simulink model "Total_B2B"  (R2018a)
settings: Solver=ode8  StartTime=0.0  StopTime=10  FixedStep=20e-6  RelTol=1e-3
values from neighbouring files (symbols this model uses):
  A = R^2*pi    (= 24996.5217713)    [Total_init.m]    (also in Total_init_trafo.m)
  C1 = 0.0117    [Total_init.m]    (also in Total_init_trafo.m)
  C2 = 5500    [Total_init.m]    (also in Total_init_trafo.m)
  C3 = 10    [Total_init.m]    (also in Total_init_trafo.m)
  C4 = 0    [Total_init.m]    (also in Total_init_trafo.m)
  C5 = 160    [Total_init.m]    (also in Total_init_trafo.m)
  C6 = 23.38    [Total_init.m]    (also in Total_init_trafo.m)
  C_dc = 1e-2    (= 0.01)    [Total_init.m]    (also in Total_init_trafo.m)
  Cx = 0    [Total_init.m]    (also in Total_init_trafo.m)
  Ir = 2*Pr/(3*Er*cosphi)    (= 2057.61316872)    [Total_init.m]    (also in Total_init_trafo.m)
  J = 12.8e6    (= 12800000)    [Total_init.m]    (also in Total_init_trafo.m)
  Jr = 3*m*r^2    (= 105248711.1)    [Total_init.m]    (also in Total_init_trafo.m)
  KI_d = KP_d*Rs/Ld    (= 1454)    [Total_init.m]    (also in Total_init_trafo.m)
  KP_d = 50    [Total_init.m]    (also in Total_init_trafo.m)
  KP_g = 5    [Total_init.m]    (also in Total_init_trafo.m)
  KP_gv = 5    [Total_init.m]    (also in Total_init_trafo.m)
  lambda_m = Er/(om_r*p)    (= 21.4859173174)    [Total_init.m]    (also in Total_init_trafo.m)
  lambda_opt = 9.35    [Total_init.m]    (also in Total_init_trafo.m)
  Ld = 0.005    [Total_init.m]    (also in Total_init_trafo.m)
  Lg = 1e-3    (= 0.001)    [Total_init.m]    (also in Total_init_trafo.m)
  Linvmat = Lmat^(-1)    [Total_init.m]    (also in Total_init_trafo.m)
  Lq = 0.005    [Total_init.m]    (also in Total_init_trafo.m)
  om0 = om_r    (= 1.0471975512)    [Total_init.m]    (also in Total_init_trafo.m)
  om_g = 100*pi    (= 314.159265359)    [Total_init.m]    (also in Total_init_trafo.m)
  om_r = 10/60*2*pi    (= 1.0471975512)    [Total_init.m]    (also in Total_init_trafo.m)
  p = 160    [Total_init.m]    (also in Total_init_trafo.m)
  Pr = 10e6    (= 10000000)    [Total_init.m]    (also in Total_init_trafo.m)
  psi0 = Lmat*I0'+psif    [Total_init.m]    (also in Total_init_trafo.m)
  psif = [lambda_m; 0]    [Total_init.m]    (also in Total_init_trafo.m)
  R = 89.2    [Total_init.m]    (also in Total_init_trafo.m)
  R_cs = 1e9    (= 1000000000)    [Total_init.m]    (also in Total_init_trafo.m)
  R_dc = 1e-3    (= 0.001)    [Total_init.m]    (also in Total_init_trafo.m)
  Rg = 1e-6    (= 1e-06)    [Total_init.m]    (also in Total_init_trafo.m)
  rho = 1.225    [Total_init.m]    (also in Total_init_trafo.m)
  Rmat = [Rs 0;         0 Rs]    [Total_init.m]    (also in Total_init_trafo.m)
  Rs = 0.1454    [Total_init.m]    (also in Total_init_trafo.m)
  ts = 0.0001    [Total_init.m]    (also in Total_init_trafo.m)
  Vac = 4000    [Total_init.m]    (also in Total_init_trafo.m)
  Vdc = Vac*sqrt(3)    [Total_init.m]    (also in Total_init_trafo.m)
  Vgsc = Vac    (= 4000)    [Total_init.m]    (also in Total_init_trafo.m)
libraries: powerlib x17, simulink x9
(part 1 of 2)
settings Model: Creator=chiel  LastModifiedBy=chiel
settings CodeAppCC: StateflowObjectComments=on

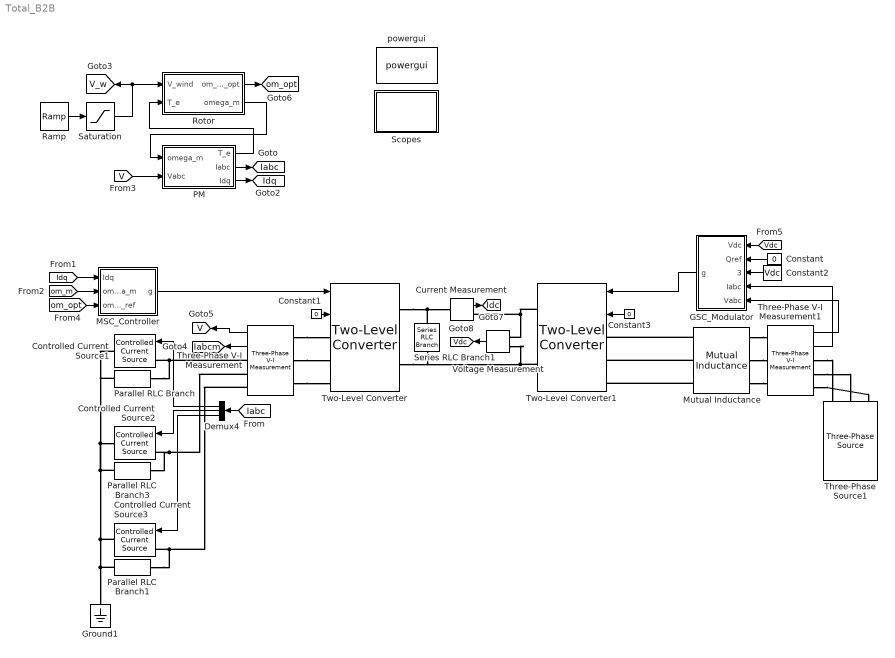
== system Total_B2B ==
  Constant : Constant  Value=0
  Constant1 : Constant  Value=0
  Constant2 : Constant  Value=Vdc
  Constant3 : Constant  Value=0
  Controlled Current Source1 : powerlib/Electrical Sources/Controlled Current Source  Initialize=on  Source_Type=AC  Amplitude=0  Phase=0  Frequency=0  Measurements=None
  Controlled Current Source2 : powerlib/Electrical Sources/Controlled Current Source  Initialize=on  Source_Type=AC  Amplitude=0  Phase=0  Frequency=0  Measurements=None
  Controlled Current Source3 : powerlib/Electrical Sources/Controlled Current Source  Initialize=on  Source_Type=AC  Amplitude=0  Phase=0  Frequency=0  Measurements=None
  Current Measurement : powerlib/Measurements/Current Measurement  PhasorSimulation=off  OutputType=Complex  PSBequivalent=0
  Demux4 : Demux  Outputs=3
  GSC_Modulator : Subsystem
  Ground1 : powerlib/Elements/Ground  LConnTagsString=a
  MSC_Controller : Subsystem
  Mutual Inductance : powerlib/Elements/Mutual Inductance  LConnTagsString=a|b|c  RConnTagsString=A|B|C  TypeOfMutual=Two or three windings with equal mutual terms  NumberOfWindings=3  SelfImpedance1=[Rg Lg]  SelfImpedance2=[Rg Lg]  ThreeWindings=on  SelfImpedance3=[Rg Lg]  MutualImpedance=[0 0]  InductanceMatrix="[1.0 0.9  0.9 ;  0.9 1.0  0.9;  0.9 0.9 1.0 ] * 1e-3"  ResistanceMatrix="[1.0 0.9  0.9 ;  0.9 1.0  0.9;  0.9 0.9 1.0 ]"  Measurements=None
      settings: AttributesFormatString=\n  SourceProductName=Simscape Power Systems  SourceProductBaseCode=PS
  PM : Subsystem
  Parallel RLC Branch : powerlib/Elements/Parallel RLC Branch  LConnTagsString=a  RConnTagsString=__new0  BranchType=R  Resistance=R_cs  Inductance=Lg  SetiL0=off  InitialCurrent=0  Capacitance=1e-6  Setx0=off  InitialVoltage=0  Measurements=None
  Parallel RLC Branch1 : powerlib/Elements/Parallel RLC Branch  LConnTagsString=a  RConnTagsString=__new0  BranchType=R  Resistance=R_cs  Inductance=Lg  SetiL0=off  InitialCurrent=0  Capacitance=1e-6  Setx0=off  InitialVoltage=0  Measurements=None
  Parallel RLC Branch3 : powerlib/Elements/Parallel RLC Branch  LConnTagsString=a  RConnTagsString=__new0  BranchType=R  Resistance=R_cs  Inductance=Lg  SetiL0=off  InitialCurrent=0  Capacitance=1e-6  Setx0=off  InitialVoltage=0  Measurements=None
  Ramp : simulink/Sources/Ramp  slope=0.5  start=0  InitialOutput=15
  Rotor : Subsystem
  Saturation : Saturate  UpperLimit=15
  Scopes : Subsystem
  Series RLC Branch1 : powerlib/Elements/Series RLC Branch  LConnTagsString=__new0  RConnTagsString=__new0  BranchType=RC  Resistance=R_dc  Inductance=1e-3  SetiL0=off  InitialCurrent=0  Capacitance=C_dc  Setx0=on  InitialVoltage=Vdc  Measurements=None
  Three-Phase V-I Measurement : powerlib/Measurements/Three-Phase V-I Measurement  VoltageMeasurement=phase-to-ground  SetLabelV=off  LabelV=Vabc  Vpu=off  VpuLL=off  CurrentMeasurement=yes  SetLabelI=off  LabelI=Iabc  Ipu=off  Pbase=100e6  Vbase=500e3  OutputType=Complex  PhasorSimulation=off  PSBequivalent=0
  Three-Phase V-I Measurement1 : powerlib/Measurements/Three-Phase V-I Measurement  VoltageMeasurement=phase-to-ground  SetLabelV=off  LabelV=Vabc  Vpu=off  VpuLL=off  CurrentMeasurement=yes  SetLabelI=off  LabelI=Iabc  Ipu=off  Pbase=100e6  Vbase=500e3  OutputType=Complex  PhasorSimulation=off  PSBequivalent=0
  Three-Phase Source1 : powerlib/Electrical Sources/Three-Phase Source  InternalConnection=Yg  VoltagePhases=off  Voltage=Vgsc/sqrt(2)*sqrt(3)  PhaseAngle=90  Voltage_phases=[25e3 25e3 25e3]/sqrt(3)  PhaseAngles_phases=[0 -120 +120]  Frequency=50  NonIdealSource=on  SpecifyImpedance=off  Resistance=1e-9  Inductance=1e-12  ShortCircuitLevel=100e6  BaseVoltage=Vgsc/sqrt(2)*sqrt(3)  XRratio=7  BusType=swing  Pref=10e3  Qref=0  Prefabc=[10e3, 10e3, 10e3]  Qrefabc=[0, 0, 0]  Qmin=-inf  Qmax=inf
  Two-Level Converter : powerlib/Power Electronics/Two-Level Converter  ModelType=Switching devices  Ron=1e-3  Rs=1e6  Cs=inf  Vforward=[0,0]  Ron_Diode=1e-3  Rs_Diode=1e6  Cs_Diode=inf  Vf_Diode=1e-3  Rs_CurrentSource=inf
      settings: SourceProductName=Simscape Power Systems  SourceProductBaseCode=PS
  Two-Level Converter1 : powerlib/Power Electronics/Two-Level Converter  ModelType=Switching function  Ron=1e-3  Rs=1e6  Cs=inf  Vforward=[0,0]  Ron_Diode=1e-3  Rs_Diode=1e6  Cs_Diode=inf  Vf_Diode=1e-3  Rs_CurrentSource=inf
      settings: SourceProductName=Simscape Power Systems  SourceProductBaseCode=PS
  Voltage Measurement : powerlib/Measurements/Voltage Measurement  PhasorSimulation=off  OutputType=Complex  PSBequivalent=0
  powergui : powerlib/powergui  Priority=1  SimulationMode=Discrete  SampleTime=20e-6  frequency=60  Iterations=50  frequencyindice=0  Pbase=100e6  ErrMax=1e-4  UnitsV=kV  UnitsW=MW  buscounter=0  FunctionMessages=off  echomessages=off  EnableUseOfTLC=off  CurrentSourceSwitches=off  DisableSnubberDevices=off  DisableRonSwitches=off  DisableVfSwitches=off  DisplayEquations=off  SolverType=Tustin/Backward Euler (TBE)  Interpol=off  ExternalGateDelay=off  methode=off  Ts=100  x0status=blocks  SPID=off  SwTol=0  HookPort=off  RestoreLinks=warning  ResistiveCurrentMeasurement=off  Frange=[0:2:500]  Ylog=off  Xlog=on  ShowGrid=off  save=off  variable=ZData  structure=0  ZoomFFT=off  StartTime=0.0  cycles=1  DisplayStyle=1  fundamental=60  FreqAxis=off  MaxFrequency=1000  frequencyindicesteady=1  RmsSteady=1  display=off
  tag scope: Iabc=global, Iabcm=global, Idc=global, Idq=global, V=global, V_w=global, Vdc=global, om_opt=global
  wires:
  [om_m] -> MSC_Controller/2(omega_m)
  [V] -> PM/2(Vabc)
  PM/2(Iabc) -> [Iabc]
  [Idq] -> MSC_Controller/1(Idq)
  PM/3(Idq) -> [Idq]
  Rotor/1(om_m_opt) -> [om_opt]
  [om_opt] -> MSC_Controller/3(omega_ref)
  Ramp/1 -> Saturation/1
  Saturation/1 -> Rotor/1(V_wind), [V_w]
  Three-Phase V-I Measurement/1 -> [V]
  Demux4/3 -> Controlled Current Source3/1
  Current Measurement/1 -> [Idc]
  Three-Phase V-I Measurement/2 -> [Iabcm]
  Constant1/1 -> Two-Level Converter/2
  Demux4/1 -> Controlled Current Source1/1
  Demux4/2 -> Controlled Current Source2/1
  [Iabc] -> Demux4/1
  Voltage Measurement/1 -> [Vdc]
  MSC_Controller/1(g) -> Two-Level Converter/1
  GSC_Modulator/1(g) -> Two-Level Converter1/1
  Constant3/1 -> Two-Level Converter1/2
  Constant/1 -> GSC_Modulator/2(Qref)
  [Vdc] -> GSC_Modulator/1(Vdc)
  Constant2/1 -> GSC_Modulator/3(Vdc_ref)
  Three-Phase V-I Measurement1/1 -> GSC_Modulator/5(Vabc)
  Three-Phase V-I Measurement1/2 -> GSC_Modulator/4(Iabc)
  Rotor/2(omega_m) -> PM/1(omega_m)
  PM/1(T_e) -> Rotor/2(T_e)
  connections:
  Controlled Current Source1/RConn1 -- Parallel RLC Branch/LConn1 -- Controlled Current Source2/RConn1 -- Parallel RLC Branch3/LConn1 -- Controlled Current Source3/RConn1 -- Ground1/LConn1 -- Parallel RLC Branch1/LConn1
  Series RLC Branch1/LConn1 -- Two-Level Converter/RConn1 -- Current Measurement/LConn1
  Voltage Measurement/LConn2 -- Two-Level Converter/RConn2 -- Series RLC Branch1/RConn1 -- Two-Level Converter1/RConn2
  Two-Level Converter1/RConn1 -- Current Measurement/RConn1 -- Voltage Measurement/LConn1
  Three-Phase V-I Measurement/LConn2 -- Two-Level Converter/LConn2
  Three-Phase V-I Measurement/RConn1 -- Parallel RLC Branch/RConn1 -- Controlled Current Source1/LConn1
  Three-Phase V-I Measurement/RConn2 -- Parallel RLC Branch3/RConn1 -- Controlled Current Source2/LConn1
  Three-Phase V-I Measurement/LConn3 -- Two-Level Converter/LConn3
  Three-Phase V-I Measurement/LConn1 -- Two-Level Converter/LConn1
  Three-Phase V-I Measurement/RConn3 -- Parallel RLC Branch1/RConn1 -- Controlled Current Source3/LConn1
  Three-Phase V-I Measurement1/RConn2 -- Three-Phase Source1/RConn2
  Three-Phase V-I Measurement1/RConn3 -- Three-Phase Source1/RConn3
  Three-Phase V-I Measurement1/RConn1 -- Three-Phase Source1/RConn1
  Mutual Inductance/LConn1 -- Two-Level Converter1/LConn1
  Mutual Inductance/LConn2 -- Two-Level Converter1/LConn2
  Mutual Inductance/LConn3 -- Two-Level Converter1/LConn3
  Mutual Inductance/RConn1 -- Three-Phase V-I Measurement1/LConn1
  Mutual Inductance/RConn2 -- Three-Phase V-I Measurement1/LConn2
  Mutual Inductance/RConn3 -- Three-Phase V-I Measurement1/LConn3

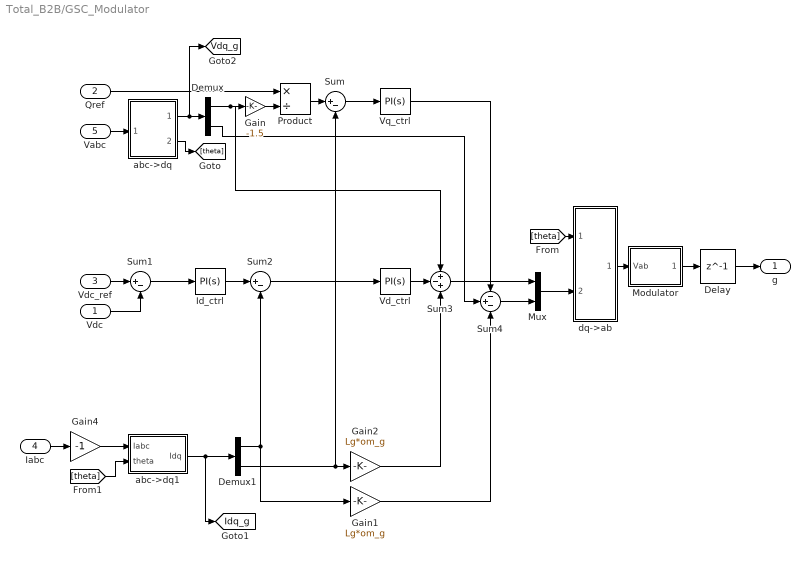
== system Total_B2B/GSC_Modulator ==
  Vdc : Inport
  Qref : Inport  Port=2
  Vdc_ref : Inport  Port=3
  Iabc : Inport  Port=4
  Vabc : Inport  Port=5
  Delay : Delay  DelayLength=1
  Demux : Demux  Outputs=2
  Demux1 : Demux  Outputs=2
  Gain : Gain  Gain=-1.5
  Gain1 : Gain  Gain=Lg*om_g
  Gain2 : Gain  Gain=Lg*om_g
  Gain4 : Gain  Gain=-1
  Id_ctrl : simulink/Continuous/PID Controller  Controller=PI  TimeDomain=Continuous-time  SampleTime=-1  IntegratorMethod=Forward Euler  FilterMethod=Forward Euler  Form=Parallel  UseFilter=on  ControllerParametersSource=internal  P=KP_gv  I=0  D=0  N=100  InitialConditionSource=internal  InitialConditionForIntegrator=0  InitialConditionForFilter=0  ExternalReset=none  LimitOutput=on  UpperSaturationLimit=Ir  LowerSaturationLimit=-Ir  LinearizeAsGain=on  AntiWindupMode=clamping  Kb=1  TrackingMode=off  Kt=1  PParamMin=[]  PParamMax=[]  IParamMin=[]  IParamMax=[]  DParamMin=[]  DParamMax=[]  NParamMin=[]  NParamMax=[]  KbParamMin=[]  KbParamMax=[]  KtParamMin=[]  KtParamMax=[]  POutMin=[]  POutMax=[]  IOutMin=[]  IOutMax=[]  DOutMin=[]  DOutMax=[]  NOutMin=[]  NOutMax=[]  KbOutMin=[]  KbOutMax=[]  KtOutMin=[]  KtOutMax=[]  IntegratorOutMin=[]  IntegratorOutMax=[]  FilterOutMin=[]  FilterOutMax=[]  SumOutMin=[]  SumOutMax=[]  SumI1OutMin=[]  SumI1OutMax=[]  SumI2OutMin=[]  SumI2OutMax=[]  SumI3OutMin=[]  SumI3OutMax=[]  SumDOutMin=[]  SumDOutMax=[]  SaturationOutMin=[]  SaturationOutMax=[]  IntegratorContinuousStateAttributes=''  IntegratorStateMustResolveToSignalObject=off  IntegratorRTWStateStorageClass=Auto  FilterContinuousStateAttributes=''  FilterStateMustResolveToSignalObject=off  FilterRTWStateStorageClass=Auto  DifferentiatorICPrevScaledInput=0  DifferentiatorOutMin=[]  DifferentiatorOutMax=[]  FilterDiffOutCoefMin=[]  FilterDiffOutCoefMax=[]  SumDenOutMin=[]  SumDenOutMax=[]  SumNumOutMin=[]  SumNumOutMax=[]  ReciprocalOutMin=[]  ReciprocalOutMax=[]  DivideOutMin=[]  DivideOutMax=[]  TunerSelectOption=Transfer Function Based (PID Tuner App)
  Modulator : Subsystem  mask{Fs=1/ts}
      mask prompts: Fs "Switching Frequency"
      mask DialogControl DescGroupVar Prompt: Swiching Parameters
  Mux : Mux  Inputs=2
  Product : Product  Inputs=*/
  Sum : Sum  Inputs=|+-
  Sum1 : Sum  Inputs=|+-
  Sum2 : Sum  Inputs=|+-
  Sum3 : Sum  Inputs=+-+
  Sum4 : Sum  Inputs=-+-
  Vd_ctrl : simulink/Continuous/PID Controller  Controller=PI  TimeDomain=Continuous-time  SampleTime=-1  IntegratorMethod=Forward Euler  FilterMethod=Forward Euler  Form=Parallel  UseFilter=on  ControllerParametersSource=internal  P=KP_g  I=0  D=0  N=100  InitialConditionSource=internal  InitialConditionForIntegrator=0  InitialConditionForFilter=0  ExternalReset=none  LimitOutput=on  UpperSaturationLimit=Vgsc  LowerSaturationLimit=-Vgsc  LinearizeAsGain=on  AntiWindupMode=clamping  Kb=1  TrackingMode=off  Kt=1  PParamMin=[]  PParamMax=[]  IParamMin=[]  IParamMax=[]  DParamMin=[]  DParamMax=[]  NParamMin=[]  NParamMax=[]  KbParamMin=[]  KbParamMax=[]  KtParamMin=[]  KtParamMax=[]  POutMin=[]  POutMax=[]  IOutMin=[]  IOutMax=[]  DOutMin=[]  DOutMax=[]  NOutMin=[]  NOutMax=[]  KbOutMin=[]  KbOutMax=[]  KtOutMin=[]  KtOutMax=[]  IntegratorOutMin=[]  IntegratorOutMax=[]  FilterOutMin=[]  FilterOutMax=[]  SumOutMin=[]  SumOutMax=[]  SumI1OutMin=[]  SumI1OutMax=[]  SumI2OutMin=[]  SumI2OutMax=[]  SumI3OutMin=[]  SumI3OutMax=[]  SumDOutMin=[]  SumDOutMax=[]  SaturationOutMin=[]  SaturationOutMax=[]  IntegratorContinuousStateAttributes=''  IntegratorStateMustResolveToSignalObject=off  IntegratorRTWStateStorageClass=Auto  FilterContinuousStateAttributes=''  FilterStateMustResolveToSignalObject=off  FilterRTWStateStorageClass=Auto  DifferentiatorICPrevScaledInput=0  DifferentiatorOutMin=[]  DifferentiatorOutMax=[]  FilterDiffOutCoefMin=[]  FilterDiffOutCoefMax=[]  SumDenOutMin=[]  SumDenOutMax=[]  SumNumOutMin=[]  SumNumOutMax=[]  ReciprocalOutMin=[]  ReciprocalOutMax=[]  DivideOutMin=[]  DivideOutMax=[]  TunerSelectOption=Transfer Function Based (PID Tuner App)
  Vq_ctrl : simulink/Continuous/PID Controller  Controller=PI  TimeDomain=Continuous-time  SampleTime=-1  IntegratorMethod=Forward Euler  FilterMethod=Forward Euler  Form=Parallel  UseFilter=on  ControllerParametersSource=internal  P=KP_g  I=0  D=0  N=100  InitialConditionSource=internal  InitialConditionForIntegrator=0  InitialConditionForFilter=0  ExternalReset=none  LimitOutput=on  UpperSaturationLimit=Vgsc  LowerSaturationLimit=-Vgsc  LinearizeAsGain=on  AntiWindupMode=none  Kb=1  TrackingMode=off  Kt=1  PParamMin=[]  PParamMax=[]  IParamMin=[]  IParamMax=[]  DParamMin=[]  DParamMax=[]  NParamMin=[]  NParamMax=[]  KbParamMin=[]  KbParamMax=[]  KtParamMin=[]  KtParamMax=[]  POutMin=[]  POutMax=[]  IOutMin=[]  IOutMax=[]  DOutMin=[]  DOutMax=[]  NOutMin=[]  NOutMax=[]  KbOutMin=[]  KbOutMax=[]  KtOutMin=[]  KtOutMax=[]  IntegratorOutMin=[]  IntegratorOutMax=[]  FilterOutMin=[]  FilterOutMax=[]  SumOutMin=[]  SumOutMax=[]  SumI1OutMin=[]  SumI1OutMax=[]  SumI2OutMin=[]  SumI2OutMax=[]  SumI3OutMin=[]  SumI3OutMax=[]  SumDOutMin=[]  SumDOutMax=[]  SaturationOutMin=[]  SaturationOutMax=[]  IntegratorContinuousStateAttributes=''  IntegratorStateMustResolveToSignalObject=off  IntegratorRTWStateStorageClass=Auto  FilterContinuousStateAttributes=''  FilterStateMustResolveToSignalObject=off  FilterRTWStateStorageClass=Auto  DifferentiatorICPrevScaledInput=0  DifferentiatorOutMin=[]  DifferentiatorOutMax=[]  FilterDiffOutCoefMin=[]  FilterDiffOutCoefMax=[]  SumDenOutMin=[]  SumDenOutMax=[]  SumNumOutMin=[]  SumNumOutMax=[]  ReciprocalOutMin=[]  ReciprocalOutMax=[]  DivideOutMin=[]  DivideOutMax=[]  TunerSelectOption=Transfer Function Based (PID Tuner App)
  abc->dq : Subsystem
  abc->dq1 : Subsystem
  dq->ab : Subsystem
  g : Outport
  tag scope: Idq_g=global, Vdq_g=global
  wires:
  Vabc/1 -> abc->dq/1(Vabc)
  Iabc/1 -> Gain4/1
  abc->dq/1(Vdq) -> [Vdq_g], Demux/1
  abc->dq1/1(Idq) -> [Idq_g], Demux1/1
  Gain/1 -> Product/2
  Qref/1 -> Product/1
  Demux1/2 -> Gain2/1, Sum/2
  Vdc/1 -> Sum1/2
  Sum1/1 -> Id_ctrl/1
  Demux1/1 -> Sum2/2, Gain1/1
  Vd_ctrl/1 -> Sum3/2
  Vq_ctrl/1 -> Sum4/1
  Mux/1 -> dq->ab/2(Vdq)
  abc->dq/2(theta) -> [theta]
  dq->ab/1(Vab) -> Modulator/1(Vab)
  Modulator/1(Out1) -> Delay/1
  Delay/1 -> g/1
  Sum/1 -> Vq_ctrl/1
  Product/1 -> Sum/1
  Sum2/1 -> Vd_ctrl/1
  Demux/1 -> Sum3/1, Gain/1
  Gain2/1 -> Sum3/3
  Sum4/1 -> Mux/2
  Demux/2 -> Sum4/2
  Gain1/1 -> Sum4/3
  Vdc_ref/1 -> Sum1/1
  Id_ctrl/1 -> Sum2/1
  Sum3/1 -> Mux/1
  Gain4/1 -> abc->dq1/1(Iabc)
  [theta] -> dq->ab/1(theta)
  [theta] -> abc->dq1/2(theta)

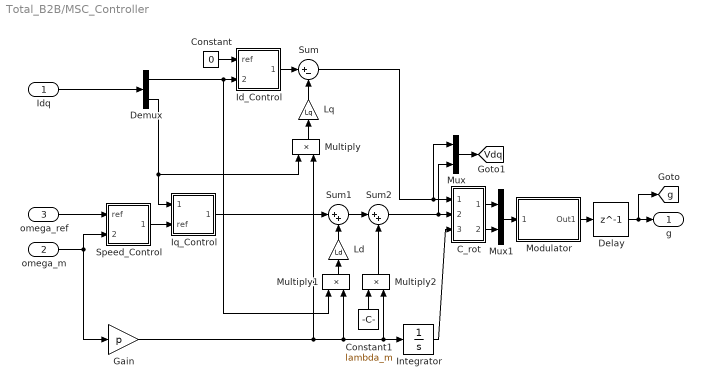
== system Total_B2B/MSC_Controller ==
  Idq : Inport
  omega_m : Inport  Port=2
  omega_ref : Inport  Port=3
  C_rot : Subsystem
  Constant : Constant  Value=0
  Constant1 : Constant  Value=lambda_m
  Delay : Delay  DelayLength=1
  Demux : Demux  Outputs=2
  Gain : Gain  Gain=p
  Id_Control : Subsystem
  Integrator : Integrator
  Iq_Control : Subsystem
  Ld : Gain  Gain=Ld
  Lq : Gain  Gain=Lq
  Modulator : Subsystem  mask{Fs=1/ts}
      mask prompts: Fs "Switching Frequency"
      mask DialogControl DescGroupVar Prompt: Swiching Parameters
  Multiply : Product
  Multiply1 : Product
  Multiply2 : Product
  Mux : Mux  Inputs=2
  Mux1 : Mux  Inputs=2
  Speed_Control : Subsystem
  Sum : Sum  Inputs=|+-
  Sum1 : Sum  Inputs=|++
  Sum2 : Sum  Inputs=|++
  g : Outport
  tag scope: Vdq=global, g=global
  wires:
  Constant/1 -> Id_Control/1(ref)
  Demux/2 -> Multiply/1, Iq_Control/1(real)
  Demux/1 -> Multiply1/1, Id_Control/2(real)
  Sum2/1 -> Mux/2, C_rot/2(in_2)
  Idq/1 -> Demux/1
  Delay/1 -> g/1, [g]
  Gain/1 -> Multiply/2, Multiply1/2, Integrator/1, Multiply2/2
  Integrator/1 -> C_rot/3(in_3)
  omega_m/1 -> Speed_Control/2(real), Gain/1
  Speed_Control/1(out) -> Iq_Control/2(ref)
  C_rot/1(out_1) -> Mux1/1
  Mux1/1 -> Modulator/1(v_albe)
  C_rot/2(out_2) -> Mux1/2
  Modulator/1(Out1) -> Delay/1
  Id_Control/1(out) -> Sum/1
  Multiply/1 -> Lq/1
  Lq/1 -> Sum/2
  Iq_Control/1(out) -> Sum1/1
  Multiply1/1 -> Ld/1
  Ld/1 -> Sum1/2
  Sum1/1 -> Sum2/1
  Multiply2/1 -> Sum2/2
  Constant1/1 -> Multiply2/1
  Sum/1 -> Mux/1, C_rot/1(in_1)
  Mux/1 -> [Vdq]
  omega_ref/1 -> Speed_Control/1(ref)

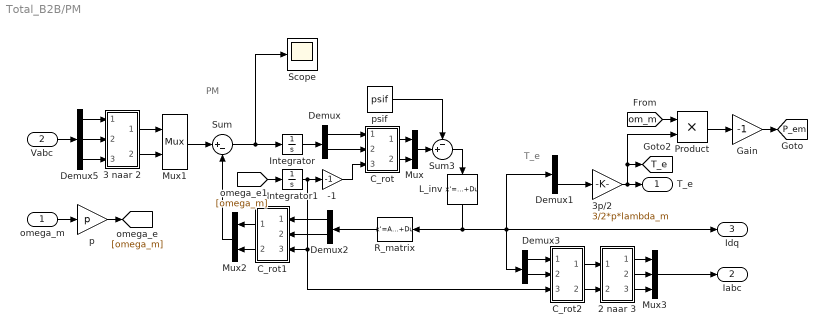
== system Total_B2B/PM ==
  note: T_e
  note: PM
  omega_m : Inport
  Vabc : Inport  Port=2
  -1 : Gain  Gain=-1  SaturateOnIntegerOverflow=on  OutDataTypeStr=Inherit: Same as input  ParamDataTypeStr=Inherit: Same as input
  2 naar 3 : Subsystem
  3 naar 2 : Subsystem
  3p/2 : Gain  Gain=3/2*p*lambda_m
  C_rot : Subsystem
  C_rot1 : Subsystem
  C_rot2 : Subsystem
  Demux{,1..3} (4 alike) : Demux  Outputs=2
  Demux5 : Demux  Outputs=3
  Gain : Gain  Gain=-1
  Integrator : Integrator  InitialCondition=psi0
  Integrator1 : Integrator
  L_inv : StateSpace  A=[]  B=[]  C=[]  D=K  InitialCondition=0  mask(Matrix gain){K=Linvmat}
      mask prompts: K "Gain matrix:"
      mask help: Matrix Gain.
      mask Help: Multiplies input vector by entered matrix to produce output vector (y=Au).
      mask Display: disp('K')
  Mux : Mux  Inputs=2
  Mux1 : Mux  Inputs=2
  Mux2 : Mux  Inputs=2
  Mux3 : Mux  Inputs=3
  Product : Product
  R_matrix : StateSpace  A=[]  B=[]  C=[]  D=K  InitialCondition=0  mask(Matrix gain){K=Rmat}
      mask prompts: K "Gain matrix:"
      mask help: Matrix Gain.
      mask Help: Multiplies input vector by entered matrix to produce output vector (y=Au).
      mask Display: disp('K')
  Scope : Scope
  Sum : Sum  Inputs=|+-
  Sum3 : Sum  Inputs=-+|
  "p " : Gain  Gain=p
  psif : Constant  Value=psif
  T_e : Outport
  Iabc : Outport  Port=2
  Idq : Outport  Port=3
  tag scope: P_em=global, T_e=global
  wires:
  Mux/1 -> Sum3/2
  C_rot1/1(out_1) -> Mux2/1
  psif/1 -> Sum3/1
  Integrator1/1 -> C_rot1/3(in_3), C_rot2/3(in_3), -1/1
  Demux/2 -> C_rot/2(in_2)
  Sum3/1 -> L_inv/1
  C_rot1/2(out_2) -> Mux2/2
  "p "/1 -> [omega_m]
  Demux/1 -> C_rot/1(in_1)
  R_matrix/1 -> Demux2/1
  Demux3/1 -> C_rot2/1(in_1)
  C_rot2/2(out_2) -> 2 naar 3/2(in_2)
  C_rot2/1(out_1) -> 2 naar 3/1(in_1)
  Mux2/1 -> Sum/2
  Mux1/1 -> Sum/1
  C_rot/2(out_2) -> Mux/2
  3 naar 2/2(out_2) -> Mux1/2
  3p/2/1 -> [T_e], Product/2, T_e/1
  3 naar 2/1(out_1) -> Mux1/1
  -1/1 -> C_rot/3(in_3)
  Demux1/2 -> 3p/2/1
  Demux2/1 -> C_rot1/1(in_1)
  Demux3/2 -> C_rot2/2(in_2)
  C_rot/1(out_1) -> Mux/1
  Demux2/2 -> C_rot1/2(in_2)
  Integrator/1 -> Demux/1
  L_inv/1 -> Demux3/1, Idq/1, Demux1/1, R_matrix/1
  Sum/1 -> Scope/1, Integrator/1
  [omega_m] -> Integrator1/1
  Demux5/1 -> 3 naar 2/1(in_1)
  Demux5/2 -> 3 naar 2/2(in_2)
  Demux5/3 -> 3 naar 2/3(in_3)
  Vabc/1 -> Demux5/1
  omega_m/1 -> "p "/1
  2 naar 3/1(out_1) -> Mux3/1
  2 naar 3/2(out_2) -> Mux3/2
  2 naar 3/3(out_3) -> Mux3/3
  Mux3/1 -> Iabc/1
  [om_m] -> Product/1
  Product/1 -> Gain/1
  Gain/1 -> [P_em]

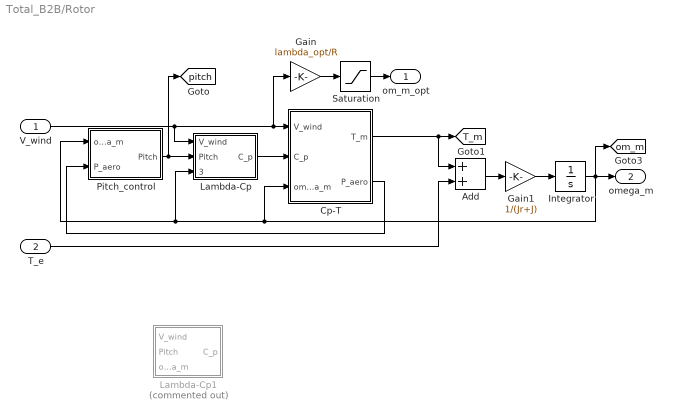
== system Total_B2B/Rotor ==
  V_wind : Inport
  T_e : Inport  Port=2
  Add : Sum
  Cp-T : Subsystem
  Gain : Gain  Gain=lambda_opt/R
  Gain1 : Gain  Gain=1/(Jr+J)
  Integrator : Integrator  InitialCondition=om0
  Lambda-Cp : Subsystem
  Lambda-Cp1 : Subsystem  Commented=on
  Pitch_control : Subsystem
  Saturation : Saturate  UpperLimit=om_r  LowerLimit=-om_r
  om_m_opt : Outport
  omega_m : Outport  Port=2
  tag scope: T_m=global, om_m=global, pitch=global
  wires:
  Integrator/1 -> Pitch_control/1(omega_m), Lambda-Cp/3(omega_m), Cp-T/3(omega_m), [om_m], omega_m/1
  Lambda-Cp/1(C_p) -> Cp-T/2(C_p)
  V_wind/1 -> Lambda-Cp/1(V_wind), Gain/1, Cp-T/1(V_wind)
  Gain/1 -> Saturation/1
  Pitch_control/1(Pitch) -> Lambda-Cp/2(Pitch), [pitch]
  Saturation/1 -> om_m_opt/1
  Cp-T/2(P_aero) -> Pitch_control/2(P_aero)
  Gain1/1 -> Integrator/1
  Cp-T/1(T_m) -> Add/1, [T_m]
  Add/1 -> Gain1/1
  T_e/1 -> Add/2

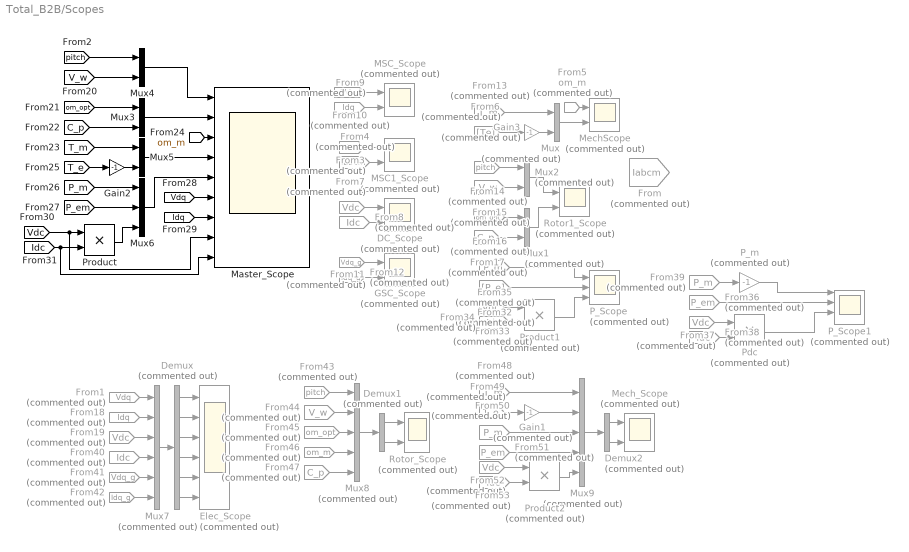
== system Total_B2B/Scopes ==
  DC_Scope : Scope  Commented=on  NumInputPorts=2
  Demux : Demux  Commented=on  Outputs=[2 2 1 1 2 2]
  Demux1 : Demux  Commented=on  Outputs=[2 3]
  Demux2 : Demux  Commented=on  Outputs=[2 3]
  Elec_Scope : Scope  Commented=on  NumInputPorts=6
  From : From  Commented=on  GotoTag=Iabcm  TagVisibility=global
  From1 : From  Commented=on  GotoTag=Vdq  TagVisibility=global
  From10 : From  Commented=on  GotoTag=Vdq  TagVisibility=global
  From11 : From  Commented=on  GotoTag=Vdq_g  TagVisibility=global
  From12 : From  Commented=on  GotoTag=Idq_g  TagVisibility=global
  From13 : From  Commented=on  GotoTag=T_m  TagVisibility=global
  From14 : From  Commented=on  GotoTag=pitch  TagVisibility=global
  From15 : From  Commented=on  GotoTag=V_w  TagVisibility=global
  From16 : From  Commented=on  GotoTag=om_opt  TagVisibility=global
  From17 : From  Commented=on  GotoTag=C_p  TagVisibility=global
  From18 : From  Commented=on  GotoTag=Idq  TagVisibility=global
  From{7,19,33,37,52} (5 alike) : From  Commented=on  GotoTag=Vdc  TagVisibility=global
  From3 : From  Commented=on  GotoTag=V  TagVisibility=global
  From32 : From  Commented=on  GotoTag=P_e  TagVisibility=global
  From{8,34,38,40,53} (5 alike) : From  Commented=on  GotoTag=Idc  TagVisibility=global
  From35 : From  Commented=on  GotoTag=P_m  TagVisibility=global
  From36 : From  Commented=on  GotoTag=P_em  TagVisibility=global
  From39 : From  Commented=on  GotoTag=P_m  TagVisibility=global
  From4 : From  Commented=on  GotoTag=Iabcm  TagVisibility=global
  From41 : From  Commented=on  GotoTag=Vdq_g  TagVisibility=global
  From42 : From  Commented=on  GotoTag=Idq_g  TagVisibility=global
  From43 : From  Commented=on  GotoTag=pitch  TagVisibility=global
  From44 : From  Commented=on  GotoTag=V_w  TagVisibility=global
  From45 : From  Commented=on  GotoTag=om_opt  TagVisibility=global
  From46 : From  Commented=on  GotoTag=om_m  TagVisibility=global
  From47 : From  Commented=on  GotoTag=C_p  TagVisibility=global
  From48 : From  Commented=on  GotoTag=T_m  TagVisibility=global
  From49 : From  Commented=on  GotoTag=T_e  TagVisibility=global
  From5 : From  Commented=on  GotoTag=om_m  TagVisibility=global
  From50 : From  Commented=on  GotoTag=P_m  TagVisibility=global
  From51 : From  Commented=on  GotoTag=P_em  TagVisibility=global
  From6 : From  Commented=on  GotoTag=Te  TagVisibility=global
  From9 : From  Commented=on  GotoTag=Idq  TagVisibility=global
  GSC_Scope : Scope  Commented=on  NumInputPorts=2
  Gain1 : Gain  Commented=on  Gain=-1
  Gain2 : Gain  Gain=-1
  Gain3 : Gain  Commented=on  Gain=-1
  MSC1_Scope : Scope  Commented=on  NumInputPorts=2
  MSC_Scope : Scope  Commented=on  NumInputPorts=2
  Master_Scope : Scope  NumInputPorts=9
  MechScope : Scope  Commented=on  NumInputPorts=2
  Mech_Scope : Scope  Commented=on  NumInputPorts=2
  Mux : Mux  Commented=on  Inputs=2
  Mux1 : Mux  Commented=on  Inputs=2
  Mux2 : Mux  Commented=on  Inputs=2
  Mux3 : Mux  Inputs=2
  Mux4 : Mux  Inputs=2
  Mux5 : Mux  Inputs=2
  Mux6 : Mux  Inputs=3
  Mux7 : Mux  Commented=on  Inputs=[2 2 1 1 2 2]
  Mux8 : Mux  Commented=on  Inputs=5
  Mux9 : Mux  Commented=on  Inputs=5
  P_Scope : Scope  Commented=on  NumInputPorts=3
  P_Scope1 : Scope  Commented=on  NumInputPorts=4
  P_m : Gain  Commented=on  Gain=-1
  Pdc : Product  Commented=on
  Product : Product
  Product1 : Product  Commented=on
  Product2 : Product  Commented=on
  Rotor1_Scope : Scope  Commented=on  NumInputPorts=2
  Rotor_Scope : Scope  Commented=on  NumInputPorts=2
  wires:
  From4/1 -> MSC1_Scope/2
  From3/1 -> MSC1_Scope/1
  From6/1 -> Gain3/1
  From5/1 -> MechScope/1
  From8/1 -> DC_Scope/2
  From7/1 -> DC_Scope/1
  From9/1 -> MSC_Scope/2
  From10/1 -> MSC_Scope/1
  From12/1 -> GSC_Scope/2
  From11/1 -> GSC_Scope/1
  From13/1 -> Mux/1
  Mux/1 -> MechScope/2
  From16/1 -> Mux1/1
  From17/1 -> Mux1/2
  Mux1/1 -> Rotor1_Scope/2
  From14/1 -> Mux2/1
  From15/1 -> Mux2/2
  Mux2/1 -> Rotor1_Scope/1
  [om_opt] -> Mux3/1
  Mux4/1 -> Master_Scope/1
  Mux3/1 -> Master_Scope/2
  [C_p] -> Mux3/2
  [pitch] -> Mux4/1
  [V_w] -> Mux4/2
  [T_e] -> Gain2/1
  Mux5/1 -> Master_Scope/4
  [T_m] -> Mux5/1
  [om_m] -> Master_Scope/3
  [P_m] -> Mux6/1
  Mux6/1 -> Master_Scope/5
  [Idq] -> Master_Scope/7
  [Vdq] -> Master_Scope/6
  [P_em] -> Mux6/2
  [Idc] -> Master_Scope/9, Product/2
  [Vdc] -> Master_Scope/8, Product/1
  Product/1 -> Mux6/3
  From34/1 -> Product1/2
  Product1/1 -> P_Scope/3
  From33/1 -> Product1/1
  From32/1 -> P_Scope/2
  From35/1 -> P_Scope/1
  Gain2/1 -> Mux5/2
  Gain3/1 -> Mux/2
  From39/1 -> P_m/1
  From37/1 -> Pdc/1
  From38/1 -> Pdc/2
  From36/1 -> P_Scope1/2
  Pdc/1 -> P_Scope1/3
  P_m/1 -> P_Scope1/1
  From41/1 -> Mux7/5
  From42/1 -> Mux7/6
  From40/1 -> Mux7/4
  From19/1 -> Mux7/3
  From18/1 -> Mux7/2
  From1/1 -> Mux7/1
  Mux7/1 -> Demux/1
  Demux/1 -> Elec_Scope/1
  Demux/2 -> Elec_Scope/2
  Demux/3 -> Elec_Scope/3
  Demux/4 -> Elec_Scope/4
  Demux/5 -> Elec_Scope/5
  Demux/6 -> Elec_Scope/6
  From45/1 -> Mux8/3
  From44/1 -> Mux8/2
  From43/1 -> Mux8/1
  From46/1 -> Mux8/4
  From47/1 -> Mux8/5
  Mux8/1 -> Demux1/1
  Demux1/2 -> Rotor_Scope/2
  Demux1/1 -> Rotor_Scope/1
  From49/1 -> Gain1/1
  From48/1 -> Mux9/1
  From51/1 -> Mux9/4
  From53/1 -> Product2/2
  From50/1 -> Mux9/3
  From52/1 -> Product2/1
  Product2/1 -> Mux9/5
  Gain1/1 -> Mux9/2
  Mux9/1 -> Demux2/1
  Demux2/2 -> Mech_Scope/2
  Demux2/1 -> Mech_Scope/1

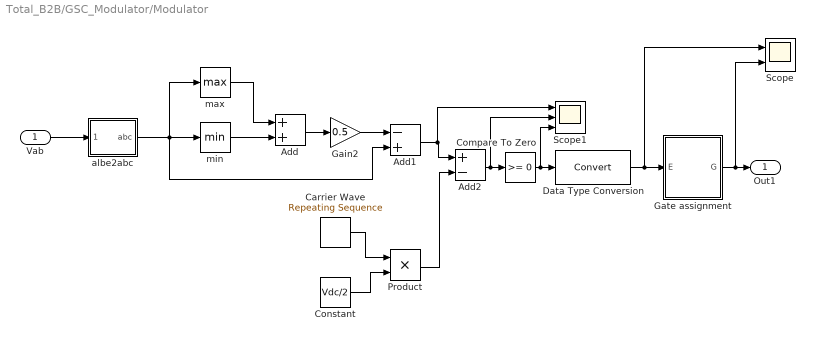
== system Total_B2B/GSC_Modulator/Modulator ==
  Vab : Inport
  Add : Sum
  Add1 : Sum  Inputs=-+
  Add2 : Sum  Inputs=+-
  Carrier Wave : simulink/Sources/Repeating Sequence  rep_seq_t=[0 0.5*ts ts]  rep_seq_y=[-1 1 -1]
  Compare To Zero : simulink/Logic and Bit Operations/Compare To Zero  relop=>=  OutDataTypeStr=boolean
  Constant : Constant  Value=Vdc/2
  Data Type Conversion : DataTypeConversion
  Gain2 : Gain  Gain=0.5
  Gate assignment : Subsystem
  Product : Product
  Scope : Scope  NumInputPorts=2
  Scope1 : Scope  NumInputPorts=3
  albe2abc : Subsystem
  max : MinMax  Function=max
  min : MinMax
  Out1 : Outport
  wires:
  Gate assignment/1(G) -> Scope/2, Out1/1
  min/1 -> Add/2
  max/1 -> Add/1
  Add/1 -> Gain2/1
  Gain2/1 -> Add1/1
  Add2/1 -> Scope1/2, Compare To Zero/1
  Constant/1 -> Product/2
  Carrier Wave/1 -> Product/1
  albe2abc/1(abc) -> Add1/2, max/1, min/1
  Product/1 -> Add2/2
  Vab/1 -> albe2abc/1(a+bj)
  Data Type Conversion/1 -> Scope/1, Gate assignment/1(E)
  Add1/1 -> Scope1/1, Add2/1
  Compare To Zero/1 -> Scope1/3, Data Type Conversion/1

== system Total_B2B/GSC_Modulator/abc->dq ==
  Vabc : Inport
  C_rot : Subsystem
  Fcn : Fcn  Expr=atan2(u(2),u(1))
  Gain : Gain  Gain=-1
  Mux : Mux  Inputs=2
  abc-ab : Subsystem
  Vdq : Outport
  theta : Outport  Port=2
  wires:
  Fcn/1 -> theta/1, Gain/1
  Gain/1 -> C_rot/2(in_3)
  Vabc/1 -> abc-ab/1(abc)
  abc-ab/1(ab) -> Fcn/1, C_rot/1(in_1)
  C_rot/1(out_1) -> Mux/1
  C_rot/2(out_2) -> Mux/2
  Mux/1 -> Vdq/1

== system Total_B2B/GSC_Modulator/abc->dq1 ==
  Iabc : Inport
  theta : Inport  Port=2
  C_rot : Subsystem
  Gain : Gain  Gain=-1
  Mux : Mux  Inputs=2
  abc-ab : Subsystem
  Idq : Outport
  wires:
  Mux/1 -> Idq/1
  abc-ab/1(ab) -> C_rot/1(in_1)
  Iabc/1 -> abc-ab/1(abc)
  C_rot/1(out_1) -> Mux/1
  theta/1 -> Gain/1
  C_rot/2(out_2) -> Mux/2
  Gain/1 -> C_rot/2(in_3)

== system Total_B2B/GSC_Modulator/dq->ab ==
  theta : Inport
  Vdq : Inport  Port=2
  C_rot : Subsystem
  Mux : Mux  Inputs=2
  Scope : Scope  NumInputPorts=3
  Vab : Outport
  wires:
  Vdq/1 -> Scope/1, C_rot/1(in_1)
  theta/1 -> Scope/2, C_rot/2(in_3)
  C_rot/1(out_1) -> Mux/1
  C_rot/2(out_2) -> Mux/2
  Mux/1 -> Scope/3, Vab/1

== system Total_B2B/MSC_Controller/C_rot ==
  in_1 : Inport
  in_2 : Inport  Port=2
  in_3 : Inport  Port=3
  Product{,1..3} (4 alike) : Product  SaturateOnIntegerOverflow=on  RndMeth=Zero  InputSameDT=on  OutDataTypeStr=Inherit: Same as first input
  Sum : Sum  Inputs=+-  SaturateOnIntegerOverflow=on  InputSameDT=on  OutDataTypeStr=Inherit: Same as first input
  Sum1 : Sum  SaturateOnIntegerOverflow=on  InputSameDT=on  OutDataTypeStr=Inherit: Same as first input
  cos : Fcn  Expr=cos(u(1))
  sin : Fcn  Expr=sin(u(1))
  out_1 : Outport
  out_2 : Outport  Port=2
  wires:
  Product2/1 -> Sum/2
  Product3/1 -> Sum1/1
  Product1/1 -> Sum/1
  Product/1 -> Sum1/2
  in_3/1 -> sin/1, cos/1
  sin/1 -> Product3/2, Product2/2
  cos/1 -> Product/2, Product1/2
  Sum/1 -> out_1/1
  Sum1/1 -> out_2/1
  in_1/1 -> Product3/1, Product1/1
  in_2/1 -> Product/1, Product2/1

== system Total_B2B/MSC_Controller/Id_Control ==
  ref : Inport
  real : Inport  Port=2
  Integrator : Integrator  LimitOutput=on  UpperSaturationLimit=Vac  LowerSaturationLimit=-Vac
  K_I : Gain  Gain=KI_d
  K_P : Gain  Gain=KP_d
  Saturation : Saturate  UpperLimit=Vac  LowerLimit=-Vac
  Sum : Sum  Inputs=|-+
  Sum1 : Sum  Inputs=|++
  TuneScope_Id : Scope  NumInputPorts=3
  out : Outport
  wires:
  ref/1 -> TuneScope_Id/1, Sum/2
  real/1 -> Sum/1, TuneScope_Id/2
  K_I/1 -> Integrator/1
  Sum/1 -> K_P/1, K_I/1
  Integrator/1 -> Sum1/1
  Sum1/1 -> Saturation/1
  K_P/1 -> Sum1/2
  Saturation/1 -> TuneScope_Id/3, out/1

== system Total_B2B/MSC_Controller/Iq_Control ==
  real : Inport
  ref : Inport  Port=2
  Integrator : Integrator  LimitOutput=on  UpperSaturationLimit=Vac  LowerSaturationLimit=-Vac
  K_I : Gain  Gain=10*Rs/Lq
  K_P : Gain  Gain=10
  Saturation : Saturate  UpperLimit=Vac  LowerLimit=-Vac
  Sum : Sum  Inputs=|-+
  Sum1 : Sum  Inputs=|++
  TuneScope_Iq : Scope  NumInputPorts=3
  out : Outport
  wires:
  real/1 -> TuneScope_Iq/1, Sum/1
  K_I/1 -> Integrator/1
  Sum/1 -> K_P/1, K_I/1
  Integrator/1 -> Sum1/1
  Sum1/1 -> Saturation/1
  K_P/1 -> Sum1/2
  Saturation/1 -> TuneScope_Iq/3, out/1
  ref/1 -> TuneScope_Iq/2, Sum/2

== system Total_B2B/MSC_Controller/Modulator ==
  v_albe : Inport
  Add : Sum
  Add1 : Sum  Inputs=-+
  Add2 : Sum  Inputs=+-
  Carrier Wave : simulink/Sources/Repeating Sequence  rep_seq_t=[0 0.5/Fs 1/Fs]  rep_seq_y=[-1 1 -1]
  Compare To Zero : simulink/Logic and Bit Operations/Compare To Zero  relop=>=  OutDataTypeStr=boolean
  Constant : Constant  Value=Vdc/2
  Data Type Conversion : DataTypeConversion
  Gain2 : Gain  Gain=0.5
  Gate assignment : Subsystem
  Product : Product
  albe2abc : Subsystem
  max : MinMax  Function=max
  min : MinMax
  Out1 : Outport
  wires:
  Gate assignment/1(G) -> Out1/1
  min/1 -> Add/2
  max/1 -> Add/1
  Add/1 -> Gain2/1
  Gain2/1 -> Add1/1
  Add2/1 -> Compare To Zero/1
  Constant/1 -> Product/2
  Carrier Wave/1 -> Product/1
  albe2abc/1(abc) -> Add1/2, min/1, max/1
  Product/1 -> Add2/2
  v_albe/1 -> albe2abc/1(a+bj)
  Compare To Zero/1 -> Data Type Conversion/1
  Data Type Conversion/1 -> Gate assignment/1(E)
  Add1/1 -> Add2/1

== system Total_B2B/MSC_Controller/Speed_Control ==
  ref : Inport
  real : Inport  Port=2
  Integrator : Integrator  LimitOutput=on  UpperSaturationLimit=Ir  LowerSaturationLimit=-Ir
  K_I : Gain  Gain=1e4
  K_P : Gain  Gain=2e4
  Saturation : Saturate  UpperLimit=Ir  LowerLimit=-Ir
  Sum : Sum  Inputs=|-+
  Sum1 : Sum  Inputs=|++
  TuneScope_w : Scope  NumInputPorts=3
  out : Outport
  wires:
  ref/1 -> Sum/2, TuneScope_w/1
  real/1 -> TuneScope_w/2, Sum/1
  K_I/1 -> Integrator/1
  Sum/1 -> K_P/1, K_I/1
  Integrator/1 -> Sum1/1
  Sum1/1 -> Saturation/1
  K_P/1 -> Sum1/2
  Saturation/1 -> TuneScope_w/3, out/1

== system Total_B2B/PM/2 naar 3 ==
  in_1 : Inport
  in_2 : Inport  Port=2
  1/w2 : Constant  Value=1/sqrt(2)
  1/w6 : Constant  Value=1/sqrt(6)
  Product : Product  SaturateOnIntegerOverflow=on  RndMeth=Zero  InputSameDT=on  OutDataTypeStr=Inherit: Same as first input
  Product1 : Product  SaturateOnIntegerOverflow=on  RndMeth=Zero  InputSameDT=on  OutDataTypeStr=Inherit: Same as first input
  Product2 : Product  SaturateOnIntegerOverflow=on  RndMeth=Zero  InputSameDT=on  OutDataTypeStr=Inherit: Same as first input
  Sum : Sum  Inputs=-+  SaturateOnIntegerOverflow=on  InputSameDT=on  OutDataTypeStr=Inherit: Same as first input
  Sum1 : Sum  Inputs=--  SaturateOnIntegerOverflow=on  InputSameDT=on  OutDataTypeStr=Inherit: Same as first input
  w2/w3 : Constant  Value=sqrt(2/3)
  out_1 : Outport
  out_2 : Outport  Port=2
  out_3 : Outport  Port=3
  wires:
  in_1/1 -> Product/2, Product1/1
  Product2/1 -> Sum1/2, Sum/2
  Product1/1 -> Sum1/1, Sum/1
  1/w2/1 -> Product2/2
  1/w6/1 -> Product1/2
  w2/w3/1 -> Product/1
  Product/1 -> out_1/1
  Sum/1 -> out_2/1
  in_2/1 -> Product2/1
  Sum1/1 -> out_3/1

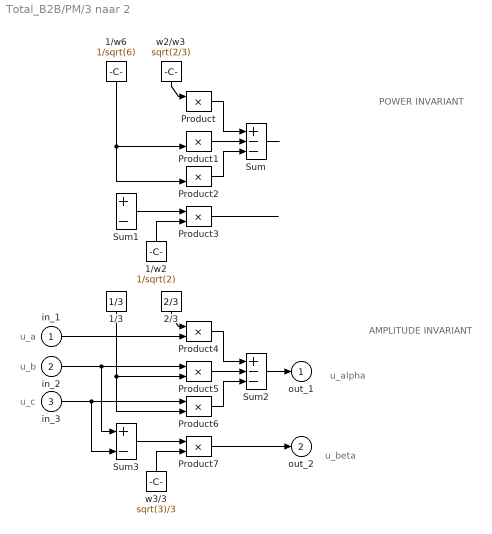
== system Total_B2B/PM/3 naar 2 ==
  note: POWER INVARIANT
  note: AMPLITUDE INVARIANT
  note: u_beta
  note: u_alpha
  note: u_a
  note: u_c
  note: u_b
  in_1 : Inport
  in_2 : Inport  Port=2
  in_3 : Inport  Port=3
  1/3 : Constant  Value=1/3
  1/w2 : Constant  Value=1/sqrt(2)
  1/w6 : Constant  Value=1/sqrt(6)
  2/3 : Constant  Value=2/3
  Product{,1..7} (8 alike) : Product  SaturateOnIntegerOverflow=on  RndMeth=Zero  InputSameDT=on  OutDataTypeStr=Inherit: Same as first input
  Sum : Sum  Inputs=+--  SaturateOnIntegerOverflow=on  InputSameDT=on  OutDataTypeStr=Inherit: Same as first input
  Sum1 : Sum  Inputs=+-  SaturateOnIntegerOverflow=on  InputSameDT=on  OutDataTypeStr=Inherit: Same as first input
  Sum2 : Sum  Inputs=+--  SaturateOnIntegerOverflow=on  InputSameDT=on  OutDataTypeStr=Inherit: Same as first input
  Sum3 : Sum  Inputs=+-  SaturateOnIntegerOverflow=on  InputSameDT=on  OutDataTypeStr=Inherit: Same as first input
  w2/w3 : Constant  Value=sqrt(2/3)
  w3/3 : Constant  Value=sqrt(3)/3
  out_1 : Outport
  out_2 : Outport  Port=2
  wires:
  1/w2/1 -> Product3/2
  Product2/1 -> Sum/3
  Sum1/1 -> Product3/1
  ? -> Sum1/2, Product2/1
  ? -> Product1/1, Sum1/1
  Product1/1 -> Sum/2
  1/w6/1 -> Product1/2, Product2/2
  w2/w3/1 -> Product/1
  Product/1 -> Sum/1
  ? -> Product/2
  Sum/1 -> ?
  Product3/1 -> ?
  in_1/1 -> Product4/2
  Product7/1 -> out_2/1
  Product6/1 -> Sum2/3
  in_3/1 -> Sum3/2, Product6/1
  2/3/1 -> Product4/1
  Product4/1 -> Sum2/1
  Product5/1 -> Sum2/2
  1/3/1 -> Product5/2, Product6/2
  in_2/1 -> Product5/1, Sum3/1
  w3/3/1 -> Product7/2
  Sum3/1 -> Product7/1
  Sum2/1 -> out_1/1

== system Total_B2B/PM/C_rot ==
  in_1 : Inport
  in_2 : Inport  Port=2
  in_3 : Inport  Port=3
  Product{,1..3} (4 alike) : Product  SaturateOnIntegerOverflow=on  RndMeth=Zero  InputSameDT=on  OutDataTypeStr=Inherit: Same as first input
  Sum : Sum  Inputs=+-  SaturateOnIntegerOverflow=on  InputSameDT=on  OutDataTypeStr=Inherit: Same as first input
  Sum1 : Sum  SaturateOnIntegerOverflow=on  InputSameDT=on  OutDataTypeStr=Inherit: Same as first input
  cos : Fcn  Expr=cos(u(1))
  sin : Fcn  Expr=sin(u(1))
  out_1 : Outport
  out_2 : Outport  Port=2
  wires:
  in_2/1 -> Product/1, Product2/1
  in_1/1 -> Product3/1, Product1/1
  Sum1/1 -> out_2/1
  Sum/1 -> out_1/1
  cos/1 -> Product/2, Product1/2
  sin/1 -> Product3/2, Product2/2
  in_3/1 -> sin/1, cos/1
  Product/1 -> Sum1/2
  Product1/1 -> Sum/1
  Product3/1 -> Sum1/1
  Product2/1 -> Sum/2

== system Total_B2B/PM/C_rot1 ==
  in_1 : Inport
  in_2 : Inport  Port=2
  in_3 : Inport  Port=3
  Product{,1..3} (4 alike) : Product  SaturateOnIntegerOverflow=on  RndMeth=Zero  InputSameDT=on  OutDataTypeStr=Inherit: Same as first input
  Sum : Sum  Inputs=+-  SaturateOnIntegerOverflow=on  InputSameDT=on  OutDataTypeStr=Inherit: Same as first input
  Sum1 : Sum  SaturateOnIntegerOverflow=on  InputSameDT=on  OutDataTypeStr=Inherit: Same as first input
  cos : Fcn  Expr=cos(u(1))
  sin : Fcn  Expr=sin(u(1))
  out_1 : Outport
  out_2 : Outport  Port=2
  wires:
  in_2/1 -> Product/1, Product2/1
  in_1/1 -> Product3/1, Product1/1
  Sum1/1 -> out_2/1
  Sum/1 -> out_1/1
  cos/1 -> Product/2, Product1/2
  sin/1 -> Product3/2, Product2/2
  in_3/1 -> sin/1, cos/1
  Product/1 -> Sum1/2
  Product1/1 -> Sum/1
  Product3/1 -> Sum1/1
  Product2/1 -> Sum/2

== system Total_B2B/PM/C_rot2 ==
  in_1 : Inport
  in_2 : Inport  Port=2
  in_3 : Inport  Port=3
  Product{,1..3} (4 alike) : Product  SaturateOnIntegerOverflow=on  RndMeth=Zero  InputSameDT=on  OutDataTypeStr=Inherit: Same as first input
  Sum : Sum  Inputs=+-  SaturateOnIntegerOverflow=on  InputSameDT=on  OutDataTypeStr=Inherit: Same as first input
  Sum1 : Sum  SaturateOnIntegerOverflow=on  InputSameDT=on  OutDataTypeStr=Inherit: Same as first input
  cos : Fcn  Expr=cos(u(1))
  sin : Fcn  Expr=sin(u(1))
  out_1 : Outport
  out_2 : Outport  Port=2
  wires:
  in_2/1 -> Product/1, Product2/1
  in_1/1 -> Product3/1, Product1/1
  Sum1/1 -> out_2/1
  Sum/1 -> out_1/1
  cos/1 -> Product/2, Product1/2
  sin/1 -> Product3/2, Product2/2
  in_3/1 -> sin/1, cos/1
  Product/1 -> Sum1/2
  Product1/1 -> Sum/1
  Product3/1 -> Sum1/1
  Product2/1 -> Sum/2

== system Total_B2B/Rotor/Cp-T ==
  V_wind : Inport
  C_p : Inport  Port=2
  omega_m : Inport  Port=3
  0.5rho*A : Gain  Gain=0.5*rho*A
  P : Product
  P_Scope : Scope  NumInputPorts=3
  T : Product  Inputs=*/
  V^3 : Product  Inputs=3
  T_m : Outport
  P_aero : Outport  Port=2
  tag scope: P_m=global
  wires:
  C_p/1 -> P_Scope/2, 0.5rho*A/1
  V_wind/1 -> V^3/3, V^3/2, V^3/1
  0.5rho*A/1 -> P/1
  V^3/1 -> P_Scope/1, P/2
  P/1 -> [P_m], P_aero/1, P_Scope/3, T/1
  omega_m/1 -> T/2
  T/1 -> T_m/1

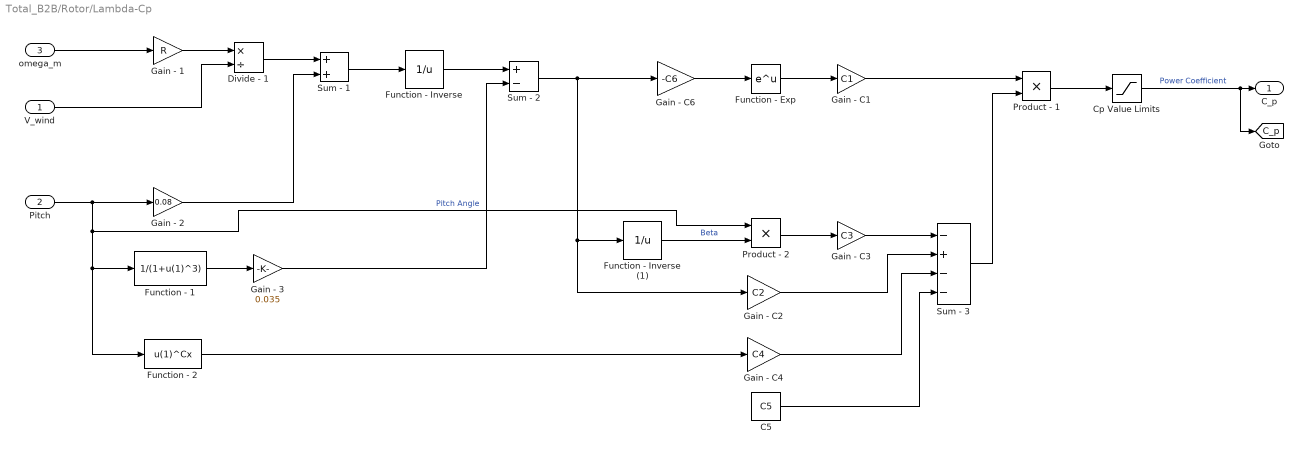
== system Total_B2B/Rotor/Lambda-Cp ==
  V_wind : Inport
  Pitch : Inport  Port=2
  omega_m : Inport  Port=3
  C5 : Constant  Value=C5
  Cp Value Limits : Saturate  LowerLimit=0
  Divide - 1 : Product  Inputs=*/
  Function - 1 : Fcn  Expr=1/(1+u(1)^3)
  Function - 2 : Fcn  Expr=u(1)^Cx
  Function - Exp : Math  SaturateOnIntegerOverflow=on
  Function - Inverse : Math  Operator=reciprocal  SaturateOnIntegerOverflow=on
  Function - Inverse (1) : Math  Operator=reciprocal  SaturateOnIntegerOverflow=on
  Gain - 1 : Gain  Gain=R
  Gain - 2 : Gain  Gain=0.08
  Gain - 3 : Gain  Gain=0.035
  Gain - C1 : Gain  Gain=C1
  Gain - C2 : Gain  Gain=C2
  Gain - C3 : Gain  Gain=C3
  Gain - C4 : Gain  Gain=C4
  Gain - C6 : Gain  Gain=-C6
  Product - 1 : Product
  Product - 2 : Product
  Sum - 1 : Sum
  Sum - 2 : Sum  Inputs=+-
  Sum - 3 : Sum  Inputs=-+--
  C_p : Outport
  tag scope: C_p=global
  wires:
  Gain - C4/1 -> Sum - 3/3
  Gain - 3/1 -> Sum - 2/2
  Product - 1/1 -> Cp Value Limits/1
  Gain - 2/1 -> Sum - 1/2
  Sum - 3/1 -> Product - 1/2
  C5/1 -> Sum - 3/4
  Sum - 2/1 -> Gain - C2/1, Function - Inverse (1)/1, Gain - C6/1
  Gain - C2/1 -> Sum - 3/2
  Function - 2/1 -> Gain - C4/1
  Gain - C3/1 -> Sum - 3/1
  Gain - C1/1 -> Product - 1/1
  Product - 2/1 -> Gain - C3/1
  Sum - 1/1 -> Function - Inverse/1
  Pitch/1 -> Gain - 2/1, Product - 2/1, Function - 2/1, Function - 1/1  "Pitch Angle"
  Divide - 1/1 -> Sum - 1/1
  Function - 1/1 -> Gain - 3/1
  V_wind/1 -> Divide - 1/2
  Gain - 1/1 -> Divide - 1/1
  Gain - C6/1 -> Function - Exp/1
  Function - Exp/1 -> Gain - C1/1
  Function - Inverse/1 -> Sum - 2/1
  Function - Inverse (1)/1 -> Product - 2/2  "Beta"
  Cp Value Limits/1 -> [C_p], C_p/1  "Power Coefficient"
  omega_m/1 -> Gain - 1/1

== system Total_B2B/Rotor/Lambda-Cp1 ==
  V_wind : Inport
  Pitch : Inport  Port=2
  omega_m : Inport  Port=3
  C_p approx : MATLAB Function  TreatAsAtomicUnit=on
  Cp_scope : Scope  NumInputPorts=3
  C_p : Outport
  tag scope: C_p=global
  wires:
  Pitch/1 -> C_p approx/2(pitch), Cp_scope/2
  C_p approx/1(C_p) -> [C_p], Cp_scope/3, C_p/1
  V_wind/1 -> Cp_scope/1, C_p approx/1(V)
  omega_m/1 -> C_p approx/3(omega)

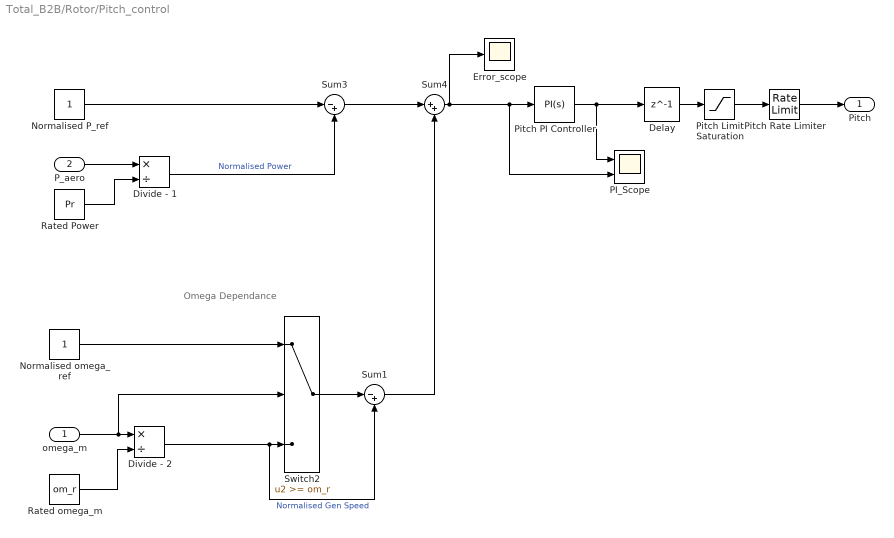
== system Total_B2B/Rotor/Pitch_control ==
  note: Omega Dependance
  omega_m : Inport
  P_aero : Inport  Port=2
  Delay : Delay  DelayLength=1
  Divide - 1 : Product  Inputs=*/
  Divide - 2 : Product  Inputs=*/
  Error_scope : Scope
  Normalised P_ref : Constant
  Normalised omega_ref : Constant
  PI_Scope : Scope  NumInputPorts=2
  Pitch Limit Saturation : Saturate  UpperLimit=90  LowerLimit=0
  Pitch PI Controller : simulink/Continuous/PID Controller  Controller=PI  TimeDomain=Continuous-time  SampleTime=-1  IntegratorMethod=Forward Euler  FilterMethod=Forward Euler  Form=Parallel  UseFilter=on  ControllerParametersSource=internal  P=154.035478691714  I=3737.60568138233  D=0  N=100  InitialConditionSource=internal  InitialConditionForIntegrator=0  InitialConditionForFilter=0  ExternalReset=none  LimitOutput=on  UpperSaturationLimit=90  LowerSaturationLimit=0  LinearizeAsGain=on  AntiWindupMode=clamping  Kb=1  TrackingMode=off  Kt=1  PParamMin=[]  PParamMax=[]  IParamMin=[]  IParamMax=[]  DParamMin=[]  DParamMax=[]  NParamMin=[]  NParamMax=[]  KbParamMin=[]  KbParamMax=[]  KtParamMin=[]  KtParamMax=[]  POutMin=[]  POutMax=[]  IOutMin=[]  IOutMax=[]  DOutMin=[]  DOutMax=[]  NOutMin=[]  NOutMax=[]  KbOutMin=[]  KbOutMax=[]  KtOutMin=[]  KtOutMax=[]  IntegratorOutMin=[]  IntegratorOutMax=[]  FilterOutMin=[]  FilterOutMax=[]  SumOutMin=[]  SumOutMax=[]  SumI1OutMin=[]  SumI1OutMax=[]  SumI2OutMin=[]  SumI2OutMax=[]  SumI3OutMin=[]  SumI3OutMax=[]  SumDOutMin=[]  SumDOutMax=[]  SaturationOutMin=[]  SaturationOutMax=[]  IntegratorContinuousStateAttributes=''  IntegratorStateMustResolveToSignalObject=off  IntegratorRTWStateStorageClass=Auto  FilterContinuousStateAttributes=''  FilterStateMustResolveToSignalObject=off  FilterRTWStateStorageClass=Auto  DifferentiatorICPrevScaledInput=0  DifferentiatorOutMin=[]  DifferentiatorOutMax=[]  FilterDiffOutCoefMin=[]  FilterDiffOutCoefMax=[]  SumDenOutMin=[]  SumDenOutMax=[]  SumNumOutMin=[]  SumNumOutMax=[]  ReciprocalOutMin=[]  ReciprocalOutMax=[]  DivideOutMin=[]  DivideOutMax=[]  TunerSelectOption=Transfer Function Based (PID Tuner App)
  Pitch Rate Limiter : RateLimiter  RisingSlewLimit=10  FallingSlewLimit=-10  SampleTimeMode=inherited
  Rated Power : Constant  Value=Pr
  Rated omega_m : Constant  Value=om_r
  Sum1 : Sum  Inputs=|-+
  Sum3 : Sum  Inputs=|-+
  Sum4 : Sum  Inputs=|++
  Switch2 : Switch  Threshold=om_r
  Pitch : Outport
  wires:
  Rated Power/1 -> Divide - 1/2
  Divide - 1/1 -> Sum3/2  "Normalised Power"
  Normalised omega_ref/1 -> Switch2/1
  Switch2/1 -> Sum1/1
  Rated omega_m/1 -> Divide - 2/2
  Divide - 2/1 -> Sum1/2, Switch2/3  "Normalised Gen Speed"
  omega_m/1 -> Switch2/2, Divide - 2/1
  Pitch Limit Saturation/1 -> Pitch Rate Limiter/1
  Pitch Rate Limiter/1 -> Pitch/1
  Normalised P_ref/1 -> Sum3/1
  P_aero/1 -> Divide - 1/1
  Sum1/1 -> Sum4/2
  Pitch PI Controller/1 -> Delay/1, PI_Scope/1
  Sum4/1 -> PI_Scope/2, Pitch PI Controller/1, Error_scope/1
  Delay/1 -> Pitch Limit Saturation/1
  Sum3/1 -> Sum4/1

== system Total_B2B/GSC_Modulator/Modulator/Gate assignment ==
  E : Inport
  Constant : Constant
  Demux : Demux  Outputs=3
  Demux1 : Demux  Outputs=3
  Mux : Mux  Inputs=6
  Sum1 : Sum  Inputs=-+|  SaturateOnIntegerOverflow=on  InputSameDT=on  OutDataTypeStr=Inherit: Same as first input
  G : Outport
  wires:
  Demux/3 -> Mux/5  "C(high)"
  Demux1/3 -> Mux/6  "C(low)"
  Mux/1 -> G/1
  Sum1/1 -> Demux1/1
  E/1 -> Sum1/1, Demux/1
  Constant/1 -> Sum1/2
  Demux/1 -> Mux/1  "A(high)"
  Demux/2 -> Mux/3  "B(high)"
  Demux1/2 -> Mux/4  "B(low)"
  Demux1/1 -> Mux/2  "A(low)"

== system Total_B2B/GSC_Modulator/Modulator/albe2abc ==
  a+bj : Inport
  Gain : Gain  Gain=[1, 0; -0.5, sqrt(3)/2; -0.5, -sqrt(3)/2 ]  Multiplication=Matrix(K*u) (u vector)
  abc : Outport
  wires:
  Gain/1 -> abc/1
  a+bj/1 -> Gain/1

== system Total_B2B/GSC_Modulator/abc->dq/C_rot ==
  in_1 : Inport
  in_3 : Inport  Port=2
  Demux : Demux  Outputs=2
  Product{,1..3} (4 alike) : Product  SaturateOnIntegerOverflow=on  RndMeth=Zero  InputSameDT=on  OutDataTypeStr=Inherit: Same as first input
  Sum : Sum  Inputs=+-  SaturateOnIntegerOverflow=on  InputSameDT=on  OutDataTypeStr=Inherit: Same as first input
  Sum1 : Sum  SaturateOnIntegerOverflow=on  InputSameDT=on  OutDataTypeStr=Inherit: Same as first input
  cos : Fcn  Expr=cos(u(1))
  sin : Fcn  Expr=sin(u(1))
  out_1 : Outport
  out_2 : Outport  Port=2
  wires:
  Demux/2 -> Product/1, Product2/1
  Demux/1 -> Product3/1, Product1/1
  Sum1/1 -> out_2/1
  Sum/1 -> out_1/1
  cos/1 -> Product/2, Product1/2
  sin/1 -> Product3/2, Product2/2
  in_3/1 -> sin/1, cos/1
  Product/1 -> Sum1/2
  Product1/1 -> Sum/1
  Product3/1 -> Sum1/1
  Product2/1 -> Sum/2
  in_1/1 -> Demux/1

== system Total_B2B/GSC_Modulator/abc->dq/abc-ab ==
  abc : Inport
  3 naar 2 : Subsystem
  Demux : Demux  Outputs=3
  Mux : Mux  Inputs=2
  ab : Outport
  wires:
  abc/1 -> Demux/1
  Demux/1 -> 3 naar 2/1(in_1)
  Demux/2 -> 3 naar 2/2(in_2)
  Demux/3 -> 3 naar 2/3(in_3)
  3 naar 2/1(out_1) -> Mux/1
  3 naar 2/2(out_2) -> Mux/2
  Mux/1 -> ab/1

== system Total_B2B/GSC_Modulator/abc->dq1/C_rot ==
  in_1 : Inport
  in_3 : Inport  Port=2
  Demux : Demux  Outputs=2
  Product{,1..3} (4 alike) : Product  SaturateOnIntegerOverflow=on  RndMeth=Zero  InputSameDT=on  OutDataTypeStr=Inherit: Same as first input
  Sum : Sum  Inputs=+-  SaturateOnIntegerOverflow=on  InputSameDT=on  OutDataTypeStr=Inherit: Same as first input
  Sum1 : Sum  SaturateOnIntegerOverflow=on  InputSameDT=on  OutDataTypeStr=Inherit: Same as first input
  cos : Fcn  Expr=cos(u(1))
  sin : Fcn  Expr=sin(u(1))
  out_1 : Outport
  out_2 : Outport  Port=2
  wires:
  Demux/2 -> Product/1, Product2/1
  Demux/1 -> Product3/1, Product1/1
  Sum1/1 -> out_2/1
  Sum/1 -> out_1/1
  cos/1 -> Product/2, Product1/2
  sin/1 -> Product3/2, Product2/2
  in_3/1 -> sin/1, cos/1
  Product/1 -> Sum1/2
  Product1/1 -> Sum/1
  Product3/1 -> Sum1/1
  Product2/1 -> Sum/2
  in_1/1 -> Demux/1

== system Total_B2B/GSC_Modulator/abc->dq1/abc-ab ==
  abc : Inport
  3 naar 2 : Subsystem
  Demux : Demux  Outputs=3
  Mux : Mux  Inputs=2
  ab : Outport
  wires:
  abc/1 -> Demux/1
  Demux/1 -> 3 naar 2/1(in_1)
  Demux/2 -> 3 naar 2/2(in_2)
  Demux/3 -> 3 naar 2/3(in_3)
  3 naar 2/1(out_1) -> Mux/1
  3 naar 2/2(out_2) -> Mux/2
  Mux/1 -> ab/1

== system Total_B2B/GSC_Modulator/dq->ab/C_rot ==
  in_1 : Inport
  in_3 : Inport  Port=2
  Demux : Demux  Outputs=2
  Product{,1..3} (4 alike) : Product  SaturateOnIntegerOverflow=on  RndMeth=Zero  InputSameDT=on  OutDataTypeStr=Inherit: Same as first input
  Sum : Sum  Inputs=+-  SaturateOnIntegerOverflow=on  InputSameDT=on  OutDataTypeStr=Inherit: Same as first input
  Sum1 : Sum  SaturateOnIntegerOverflow=on  InputSameDT=on  OutDataTypeStr=Inherit: Same as first input
  cos : Fcn  Expr=cos(u(1))
  sin : Fcn  Expr=sin(u(1))
  out_1 : Outport
  out_2 : Outport  Port=2
  wires:
  Demux/2 -> Product/1, Product2/1
  Demux/1 -> Product3/1, Product1/1
  Sum1/1 -> out_2/1
  Sum/1 -> out_1/1
  cos/1 -> Product/2, Product1/2
  sin/1 -> Product3/2, Product2/2
  in_3/1 -> sin/1, cos/1
  Product/1 -> Sum1/2
  Product1/1 -> Sum/1
  Product3/1 -> Sum1/1
  Product2/1 -> Sum/2
  in_1/1 -> Demux/1
